simulink model "SolarCellModel2"  (R2020a)
settings: Solver=VariableStepAuto  StartTime=0.0  StopTime=250  MaxStep=0.1  RelTol=1e-3  AbsTol=1e-3  EnableMultiTasking=on
PreLoadFcn:
  | irradiance = 1000;
  | temperature = 25;
StopFcn:
  | ee_addSimlogTimeStamp(bdroot)
undefined symbols (not defined in the file): Irradiance11, Irradiance21, Irradiance31, Irradiance41
libraries: fl_lib x7, nesl_utility x7, ee_lib x4, simulink x1
CloseFcn:
  | try,close(h1_ee_solar_cell),end
  | clear h1_ee_solar_cell
  | 
  | 
  | clear simlog_ee_solar_cell
  | clear logsout_ee_solar_cell
  | clear I Pmax V_Pmax idx index irradiance irradianceVec legend_info powerMat powerTable temperature temperatureVec vVec voltageTable
Description:
  | Solar Cell Power Curve
settings Model: Creator=The MathWorks, Inc.  LastModifiedBy=ASUS
settings SolverCC: AutoScaleAbsTol=off  InitialStep=0.1
settings DataIOCC: MaxDataPoints=10000  SaveFormat=Array  SaveOutput=off  SignalLogging=off  DSMLogging=off  SaveTime=off  ReturnWorkspaceOutputs=off  SignalLoggingName=logsout_ee_solar_cell  OutputOption=SpecifiedOutputTimes  OutputTimes=[0:0.5:60]
settings OptimizationCC: ExpressionDepthLimit=2147483647  LifeSpan=inf
settings DebuggingCC: UnderspecifiedInitializationDetection=Classic  MergeDetectMultiDrivingBlocksExec=none  FcnCallInpInsideContextMsg=warning  StateNameClashWarn=warning  SFUnexpectedBacktrackingDiag=warning  SFNoUnconditionalDefaultTransitionDiag=warning  SFExecutionAtInitializationDiag=none  ArithmeticOperatorsInVariantConditions=warning
settings HardwareCC: ProdBitPerPointer=32  ProdBitPerSizeT=32  ProdBitPerPtrDiffT=32  ProdLargestAtomicFloat=None  ProdIntDivRoundTo=Undefined  ProdEndianess=Unspecified  ProdWordSize=32  ProdHWDeviceType=32-bit Generic
settings ModelReferenceCC: PropagateSignalLabelsOutOfModel=off
settings SFSimCC: SimUseLocalCustomCode=off  CustomCodeUndefinedFunction=UseInterfaceOnly
settings RTWCC: RTWUseLocalCustomCode=off
settings CodeAppCC: StateflowObjectComments=on
settings GRTTargetCC: TargetLangStandard=C89/C90 (ANSI)  CombineOutputUpdateFcns=off  GRTInterface=on
settings ConfigComp: CovMetricSettings=dw  CovHtmlReporting=on  CovSaveCumulativeToWorkspaceVar=on  CovSaveSingleToWorkspaceVar=on  CovExternalEMLEnable=off  CovSFcnEnable=off
settings SimscapeCC: SimscapeLogType=all  SimscapeLogSimulationStatistics=on  SimscapeLogName=simlog_ee_solar_cell  SimscapeLogDataHistory=10000

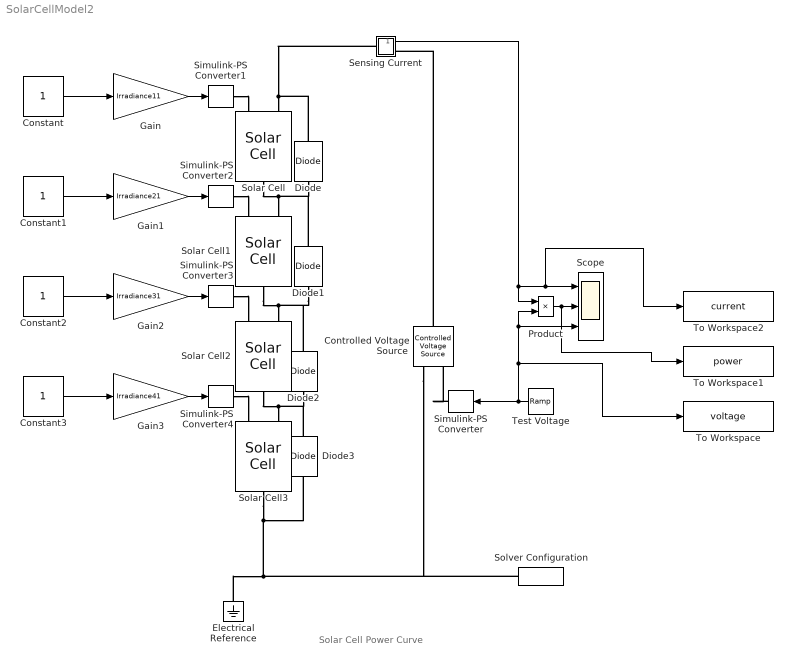
== system SolarCellModel2 ==
  note: Solar Cell Power Curve
  Constant{,1..3} (4 alike) : Constant  VectorParams1D=off  SampleTime=-1
  Controlled Voltage Source : fl_lib/Electrical/Electrical Sources/Controlled Voltage Source
      settings: SourceProductBaseCode=MT,SS
  Diode{,1..3} (4 alike) : fl_lib/Electrical/Electrical Elements/Diode  Vf=0.6 V  Ron=0.3 Ohm  Goff=1e-8 1/Ohm  i_specify=off  i_priority=None  i=0 A  i_nominal_specify=off  i_nominal_unit=A  i_nominal_value=1  v_specify=off  v_priority=None  v=0 V  v_nominal_specify=off  v_nominal_unit=V  v_nominal_value=1
  Electrical Reference : fl_lib/Electrical/Electrical Elements/Electrical Reference
      settings: SourceProductBaseCode=MT,SS
  Gain : Gain  Gain=Irradiance11
  Gain1 : Gain  Gain=Irradiance21
  Gain2 : Gain  Gain=Irradiance31
  Gain3 : Gain  Gain=Irradiance41
  Product : Product  InputSameDT=on  SaturateOnIntegerOverflow=on  OutDataTypeStr=Inherit: Same as first input
  Scope : Scope  NumInputPorts=3
  Sensing Current : Subsystem
      mask Display: disp('i')
  Simulink-PS Converter{,1..4} (5 alike) : nesl_utility/Simulink-PS Converter  PhysicalDomain=network_engine_domain  SubClassName=ps_input  LeftPortType=input  RightPortType=output  PseudoPeriodic=off  Frequencies=[]  NoiseDistribution=none  NoiseParameters=[]  Unit=1  AffineConversion=off  FilteringAndDerivatives=zero  SimscapeFilterOrder=1  InputFilterTimeConstant=0.001  UdotUserProvided=1
      settings: SourceProductBaseCode=MT,SS
  Solar Cell{,1..3} (4 alike) : ee_lib/Sources/Solar Cell  prm=3  Isc=3.8 A  Voc=0.586 V  Is=3.15e-07 A  Is2=0 A  Iph=3.80 A  Ir0=1000 W/m^2  ec=1.4  N2=2  Rs=series_resistance Ohm  Rp=parallel_resistance Ohm  N_series=700  TIPH1=0.000805 1/K  EG=1.11 eV  TXIS1=3.38  TXIS2=3  TRS1=0  TRP1=0  Tmeas=25 degC  TFIXED=temperature degC  thermal_mass=100 J/K  initial_temperature=25 degC
      settings: SourceProductBaseCode=PS
  Solver Configuration : nesl_utility/Solver Configuration  PhysicalDomain=network_engine_domain  SubClassName=solver  LeftPortType=input  RightPortType=generic  Tones=[]  Harmonics=[]  SimulateNoise=off  Profile=off  UseLocalSampling=off  EnableSwitchedLinearOptims=on  FrequencyDomain=off  UseCCode=off  RelTol=0.001  AbsTol=1e-06  MinStep=1e-09  ToWorkspace=off  RevertToSquareIcSolve=off  NumHomotopyIterations=100  PhasorMode=off  PhasorModeNumHarmonics=1  DoDC=off  ResidualTolerance=1e-9  UseLocalSolver=off  LocalSolverChoice=NE_BACKWARD_EULER_ADVANCER  LocalSolverSampleTime=0.1  DoFixedCost=off  MaxNonlinIter=3  MaxModeIter=2  LinearAlgebra=auto  EquationFormulation=NE_TIME_EF  DelaysMemoryBudget=1024  AutomaticFiltering=on  FilteringTimeConstant=0.001  PartitionStorageMethod=AS_NEEDED  PartitionMemoryBudget=1024  PartitionMethod=FAST
      settings: SourceProductBaseCode=MT,SS
  Test Voltage : simulink/Sources/Ramp  slope=500/60  start=0  InitialOutput=0
  To Workspace : ToWorkspace  VariableName=voltage  SampleTime=-1
  To Workspace1 : ToWorkspace  VariableName=power  SampleTime=-1
  To Workspace2 : ToWorkspace  VariableName=current  SampleTime=-1
  wires:
  Product/1 -> To Workspace1/1, Scope/2
  Test Voltage/1 -> Simulink-PS Converter/1, To Workspace/1, Scope/3, Product/2
  Sensing Current/1(Out1) -> Product/1, To Workspace2/1, Scope/1
  Constant/1 -> Gain/1
  Gain/1 -> Simulink-PS Converter1/1
  Gain1/1 -> Simulink-PS Converter2/1
  Constant1/1 -> Gain1/1
  Constant3/1 -> Gain3/1
  Gain3/1 -> Simulink-PS Converter4/1
  Gain2/1 -> Simulink-PS Converter3/1
  Constant2/1 -> Gain2/1
  connections:
  Simulink-PS Converter/RConn1 -- Controlled Voltage Source/RConn1
  Controlled Voltage Source/LConn1 -- Sensing Current/RConn1
  Simulink-PS Converter1/RConn1 -- Solar Cell/LConn1
  Simulink-PS Converter2/RConn1 -- Solar Cell1/LConn1
  Simulink-PS Converter4/RConn1 -- Solar Cell3/LConn1
  Simulink-PS Converter3/RConn1 -- Solar Cell2/LConn1
  Solar Cell1/RConn1 -- Diode2/RConn1 -- Diode1/LConn1 -- Solar Cell2/LConn2
  Solar Cell2/RConn1 -- Diode3/RConn1 -- Diode2/LConn1 -- Solar Cell3/LConn2
  Solar Cell/RConn1 -- Diode1/RConn1 -- Diode/LConn1 -- Solar Cell1/LConn2
  Diode/RConn1 -- Sensing Current/LConn1 -- Solar Cell/LConn2
  Solar Cell3/RConn1 -- Diode3/LConn1 -- Controlled Voltage Source/RConn2 -- Solver Configuration/RConn1 -- Electrical Reference/LConn1

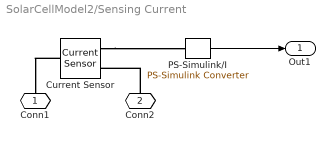
== system SolarCellModel2/Sensing Current ==
  Current Sensor : fl_lib/Electrical/Electrical Sensors/Current Sensor
      settings: SourceProductBaseCode=MT,SS
  PS-Simulink/I : nesl_utility/PS-Simulink Converter  PhysicalDomain=network_engine_domain  SubClassName=ps_output  LeftPortType=input  RightPortType=output  PseudoPeriodic=off  Frequencies=[]  Unit=1  AffineConversion=off
      settings: SourceProductBaseCode=MT,SS
  Conn1 : PMIOPort  Side=Left
  Conn2 : PMIOPort  Port=2  Side=Right
  Out1 : Outport  VectorParamsAs1DForOutWhenUnconnected=off
  wires:
  PS-Simulink/I/1 -> Out1/1
  connections:
  Current Sensor/RConn1 -- PS-Simulink/I/LConn1
  Current Sensor/LConn1 -- Conn1/RConn1
  Conn2/RConn1 -- Current Sensor/RConn2
